simulink model "Kinematic"  (R2021b)
settings: Solver=VariableStepAuto  StartTime=0.0  StopTime=100  RelTol=1e-3
undefined symbols (not defined in the file): q_init, Ts, w_I0_0, w_IB_B
libraries: sharedtransform x3
settings Model: Creator=DCLab  LastModifiedBy=DCLab

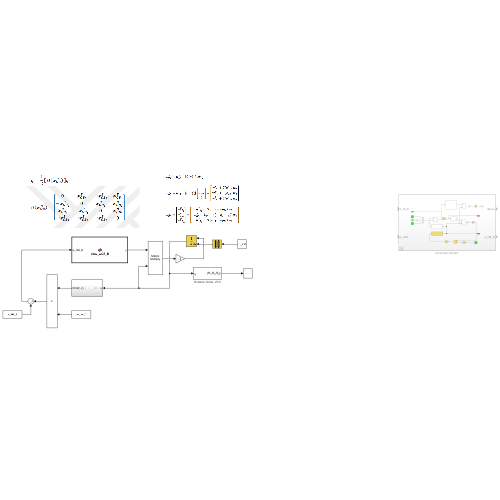
[thumbnail: Simulink's stored preview of the top-level diagram]
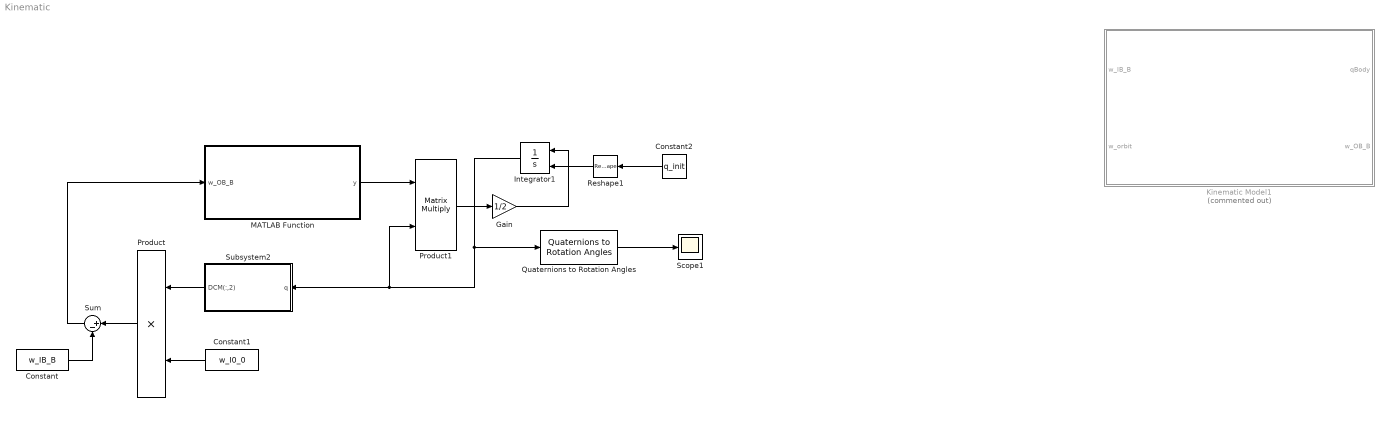
== system Kinematic ==
  Constant : Constant  Value=w_IB_B
  Constant1 : Constant  Value=w_I0_0
  Constant2 : Constant  Value=q_init
  Gain : Gain  Gain=1/2
  Integrator1 : Integrator  InitialConditionSource=external
  Kinematic Model1 : Subsystem  Commented=on
  MATLAB Function : MATLAB Function  TreatAsAtomicUnit=on
  Product : Product
  Product1 : Product  Multiplication=Matrix(*)
  Quaternions to Rotation Angles : sharedtransform/Quaternions to Rotation Angles  rotationOrder=ZYX  aMode=aMode
      settings: SourceProductBaseCode=AE,PW,DR,MT,UV,VE
  Reshape1 : Reshape  OutputDimensionality=Column vector (2-D)
  Scope1 : Scope
  Subsystem2 : Subsystem
  Sum : Sum  Inputs=|+-
  wires:
  Constant1/1 -> Product/2
  MATLAB Function/1(y) -> Product1/1
  Product1/1 -> Gain/1
  Subsystem2/1(DCM(:,2)) -> Product/1
  Product/1 -> Sum/1
  Constant/1 -> Sum/2
  Sum/1 -> MATLAB Function/1(w_OB_B)
  Quaternions to Rotation Angles/1 -> Scope1/1
  Reshape1/1 -> Integrator1/2
  Gain/1 -> Integrator1/1
  Integrator1/1 -> Product1/2, Subsystem2/1(q), Quaternions to Rotation Angles/1
  Constant2/1 -> Reshape1/1

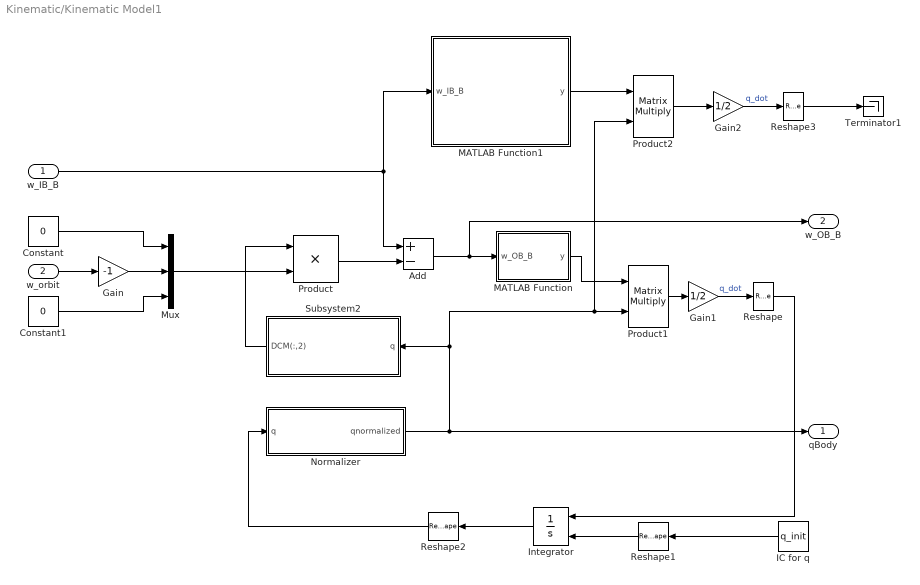
== system Kinematic/Kinematic Model1 ==
  w_IB_B : Inport
  w_orbit : Inport  Port=2
  Add : Sum  Inputs=+-
  Constant : Constant  Value=0
  Constant1 : Constant  Value=0
  Gain : Gain  Gain=-1
  Gain1 : Gain  Gain=1/2
  Gain2 : Gain  Gain=1/2
  IC for q : Constant  Value=q_init  SampleTime=Ts
  Integrator : Integrator  InitialConditionSource=external
  MATLAB Function : MATLAB Function  TreatAsAtomicUnit=on
  MATLAB Function1 : MATLAB Function  TreatAsAtomicUnit=on
  Mux : Mux  Inputs=3
  Normalizer : MATLAB Function  TreatAsAtomicUnit=on
  Product : Product
  Product1 : Product  Multiplication=Matrix(*)
  Product2 : Product  Multiplication=Matrix(*)
  Reshape{,1..3} (4 alike) : Reshape  OutputDimensionality=Column vector (2-D)
  Subsystem2 : Subsystem
  Terminator1 : Terminator
  qBody : Outport  VectorParamsAs1DForOutWhenUnconnected=off
  w_OB_B : Outport  Port=2  VectorParamsAs1DForOutWhenUnconnected=off
  wires:
  Reshape2/1 -> Normalizer/1(q)
  Product/1 -> Add/2
  Integrator/1 -> Reshape2/1
  Normalizer/1(qnormalized) -> qBody/1, Subsystem2/1(q), Product1/2, Product2/2
  IC for q/1 -> Reshape1/1
  Reshape1/1 -> Integrator/2
  Add/1 -> MATLAB Function/1(w_OB_B), w_OB_B/1
  w_orbit/1 -> Gain/1
  Mux/1 -> Product/2
  Constant/1 -> Mux/1
  Constant1/1 -> Mux/3
  Product1/1 -> Gain1/1
  MATLAB Function/1(y) -> Product1/1
  Gain1/1 -> Reshape/1  "q_dot"
  w_IB_B/1 -> MATLAB Function1/1(w_IB_B), Add/1
  Product2/1 -> Gain2/1
  MATLAB Function1/1(y) -> Product2/1
  Gain2/1 -> Reshape3/1  "q_dot"
  Subsystem2/1(DCM(:,2)) -> Product/1
  Gain/1 -> Mux/2
  Reshape/1 -> Integrator/1
  Reshape3/1 -> Terminator1/1

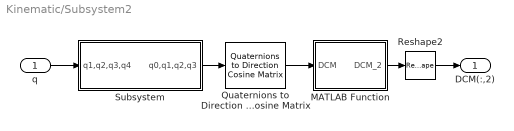
== system Kinematic/Subsystem2 ==
  q : Inport
  MATLAB Function : MATLAB Function  TreatAsAtomicUnit=on
  Quaternions to Direction Cosine Matrix : sharedtransform/Quaternions to  Direction Cosine Matrix  aMode=aMode
      settings: SourceProductBaseCode=AE,PW,DR,MT,UV,VE
  Reshape2 : Reshape  OutputDimensionality=Column vector (2-D)
  Subsystem : Subsystem
  DCM(:,2) : Outport  VectorParamsAs1DForOutWhenUnconnected=off
  wires:
  Subsystem/1(q0,q1,q2,q3) -> Quaternions to Direction Cosine Matrix/1
  q/1 -> Subsystem/1(q1,q2,q3,q4)
  Quaternions to Direction Cosine Matrix/1 -> MATLAB Function/1(DCM)
  MATLAB Function/1(DCM_2) -> Reshape2/1
  Reshape2/1 -> DCM(:,2)/1

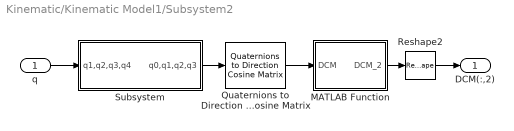
== system Kinematic/Kinematic Model1/Subsystem2 ==
  q : Inport
  MATLAB Function : MATLAB Function  TreatAsAtomicUnit=on
  Quaternions to Direction Cosine Matrix : sharedtransform/Quaternions to  Direction Cosine Matrix  aMode=aMode
      settings: SourceProductBaseCode=AE,PW,DR,MT,UV,VE
  Reshape2 : Reshape  OutputDimensionality=Column vector (2-D)
  Subsystem : Subsystem
  DCM(:,2) : Outport  VectorParamsAs1DForOutWhenUnconnected=off
  wires:
  Subsystem/1(q0,q1,q2,q3) -> Quaternions to Direction Cosine Matrix/1
  q/1 -> Subsystem/1(q1,q2,q3,q4)
  Quaternions to Direction Cosine Matrix/1 -> MATLAB Function/1(DCM)
  MATLAB Function/1(DCM_2) -> Reshape2/1
  Reshape2/1 -> DCM(:,2)/1

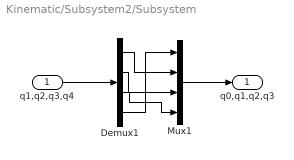
== system Kinematic/Subsystem2/Subsystem ==
  q1,q2,q3,q4 : Inport
  Demux1 : Demux
  Mux1 : Mux
  q0,q1,q2,q3 : Outport  VectorParamsAs1DForOutWhenUnconnected=off
  wires:
  Demux1/2 -> Mux1/3
  q1,q2,q3,q4/1 -> Demux1/1
  Mux1/1 -> q0,q1,q2,q3/1
  Demux1/4 -> Mux1/1
  Demux1/1 -> Mux1/2
  Demux1/3 -> Mux1/4

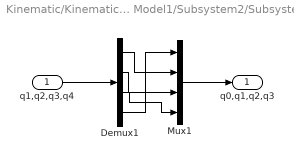
== system Kinematic/Kinematic Model1/Subsystem2/Subsystem ==
  q1,q2,q3,q4 : Inport
  Demux1 : Demux
  Mux1 : Mux
  q0,q1,q2,q3 : Outport  VectorParamsAs1DForOutWhenUnconnected=off
  wires:
  Demux1/2 -> Mux1/3
  q1,q2,q3,q4/1 -> Demux1/1
  Mux1/1 -> q0,q1,q2,q3/1
  Demux1/4 -> Mux1/1
  Demux1/1 -> Mux1/2
  Demux1/3 -> Mux1/4

== matlab function Kinematic/Subsystem2/MATLAB Function ==
  data: DCM input; DCM_2 output
function DCM_2 = fcn(DCM)
DCM_2 = DCM(:,2);
end

== matlab function Kinematic/Kinematic Model1/Subsystem2/MATLAB Function ==
  data: DCM input; DCM_2 output
function DCM_2 = fcn(DCM)
DCM_2 = DCM(:,2);
end

== matlab function Kinematic/Kinematic Model1/MATLAB Function ==
  data: w_OB_B input; y output
function y = skew_wOB_B(w_OB_B)


y = [0, w_OB_B(3,1), -w_OB_B(2,1), w_OB_B(1,1);...
    -w_OB_B(3,1), 0, w_OB_B(1,1), w_OB_B(2,1);...
     w_OB_B(2,1), -w_OB_B(1,1), 0, w_OB_B(3,1);...
    -w_OB_B(1,1), -w_OB_B(2,1), -w_OB_B(3,1), 0];
end

== matlab function Kinematic/Kinematic Model1/Normalizer ==
  data: qnormalized output; q input
function qnormalized = fcn(q)

%Normalizes the quaternion

qnormalized = q;
qs = q(4);
qv = [q(1); q(2); q(3)];

qnormalized(4)= qs /norm(q);
qnormalized(1)= qv(1)/norm(q);
qnormalized(2)= qv(2)/norm(q);
qnormalized(3)= qv(3)/norm(q);

== matlab function Kinematic/Kinematic Model1/MATLAB Function1 ==
  data: w_IB_B input; y output
function y = skew_wIB_B(w_IB_B)


y = [0, w_IB_B(3,1), -w_IB_B(2,1), w_IB_B(1,1);...
    -w_IB_B(3,1), 0, w_IB_B(1,1), w_IB_B(2,1);...
     w_IB_B(2,1), -w_IB_B(1,1), 0, w_IB_B(3,1);...
    -w_IB_B(1,1), -w_IB_B(2,1), -w_IB_B(3,1), 0];
end

== matlab function Kinematic/MATLAB Function ==
  data: w_OB_B input; y output
function y = skew_wOB_B(w_OB_B)


y = [0, w_OB_B(3,1), -w_OB_B(2,1), w_OB_B(1,1);...
    -w_OB_B(3,1), 0, w_OB_B(1,1), w_OB_B(2,1);...
     w_OB_B(2,1), -w_OB_B(1,1), 0, w_OB_B(3,1);...
    -w_OB_B(1,1), -w_OB_B(2,1), -w_OB_B(3,1), 0];
end
